simulink model "modular"  (R2013a)
settings: Solver=ode45  StartTime=0.0  StopTime=10.0  RelTol=1e-3
libraries: gated_decay_choice x1, range_choice x1, synaptic_scaling_choice x1
settings Model: Creator=Leo  LastModifiedBy=Leo

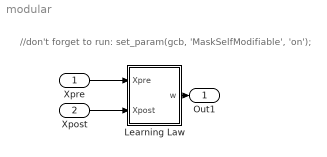
== system modular ==
  note: //don't forget to run:
      | set_param(gcb, 'MaskSelfModifiable', 'on');
  Xpre : Inport
  Xpost : Inport  Port=2
  Learning Law : Subsystem  mask{gorch_y_n=on, gated_decay=Dual OR, multdiv=Divide, synscale=Vanilla Oja, gorch_range=0, lambda1=1, lambda2=0, lambda3=0, lambda4=0, w_0=0, w0=0, alpha1=0, alpha2=0, beta=0, equ=lambda2*[Xpre*Xpost*(gorchrange)+ lambda1*(w_0-w) / ((alpha1*Xpre+alpha2*Xpost^2)*(w-w_0)) + .5lambda3*lambda4*(w_0 - w)comp(w_0,w)*(g(Xpost) - |g(Xpost)|)(g(Xpost))], extr=dg(X)/dt = s-AX, g(0) = -t, comp(w0,w) = |w0-w| <= range}
      mask prompts: gorch_y_n "Would you like a Gorch range?"; gated_decay "What kind of gated decay do you want"; multdiv "Multiply or Divide by the Gated Decay"; synscale "Synaptic Scaling"; gorch_range "Gorch Range"; lambda1 "Learning Rate (1) - Stability"; lambda2 "Learning Rate (2) - Total"; lambda3 "Learning Rate (3, Oja Specific) - Increment"; lambda4 "Learning Rate (4, Oja Specific) - Decrement"; w_0 "Range"; w0 "Initial weight"; alpha1 "Alpha 1 (Additional Parameter)"; alpha2 "Alpha 2 (Additional Parameter)"; beta "Beta (Gorch Gating Term)"; equ "Equation"; extr "Extra info"
      mask help: Make sure to hit apply after selecting your Law Type before moving on to the Law Parameters Tab.
      mask init:
      | eqw ='lambda2*[';
      | dab = gcb;
      | set_param(dab,'extr','');
      | currentVis = get_param(dab,'MaskVisibilities');
      | currentVis{12} = 'off';
      | currentVis{13} = 'off';
      | currentVis{14} = 'off';
      | 
      | if(gorch_y_n)
      |     set_param([dab '/Range'], 'BlockChoice', 'Gorch_range');
      |     currentVis{5} = 'on';
      |     eqw = [eqw 'Xpre*Xpost*(gorchrange)'];
      | else
      |     set_param([dab '/Range'], 'BlockChoice', 'Simple');
      |     currentVis{5} = 'off';
      |     eqw = [eqw 'Xpre*Xpost'];
      | end
      | 
      | eqw = [eqw '+ lambda1*(w_0-w)']
      | 
      | switch multdiv
      |     case 1 %'Multiply'
      |         set_param([dab '/TimesOrDivide'],'Inputs','**');
      |         eqw = [eqw ' * '];
      |     case 2 %'Divide'
      |         set_param([dab '/TimesOrDivide'],'Inputs','*/');
      |         eqw = [eqw ' / '];
      |     case 3 %'Inverse Divide'
      |         set_param([dab '/TimesOrDivide'],'Inputs','/*');
      |         eqw = [eqw ' \ '];
      | end
      | 
      | switch gated_decay
      |     case 1 %'Xpre'
      |         set_param([dab '/Gated Decay Choice'], 'BlockChoice', 'X_pre');
      |         eqw = [eqw 'Xpre'];
      |     case 2 %'Xpost'
      |         set_param([dab '/Gated Decay Choice'], 'BlockChoice', 'X_post');
      |         eqw = [eqw 'Xpost'];
      |     case 3 %'Gorch'
      |         set_param([dab '/Gated Decay Choice'], 'BlockChoice', 'Gorch_Gating');
      |         eqw = [eqw '(Xpost^2 * beta)'];
      |         currentVis{14} = 'on';
      |     case 4 %'Oja'
      |         set_param([dab '/Gated Decay Choice'], 'BlockChoice', 'Oja_Gating');
      |         eqw = [eqw '(Xpost^2*(w-w_0))'];
      |         currentVis{14} = 'off';
      |     case 5 %'Dual OR'
      |         set_param([dab '/Gated Decay Choice'], 'BlockChoice', 'Dual_OR');
      |         eqw = [eqw '((alpha1*Xpre+alpha2*Xpost^2)*(w-w_0))'];
      |         currentVis{12} = 'on';
      |         currentVis{13} = 'on';
      |     case 6 %'Dual AND'
      |         set_param([dab '/Gated Decay Choice'], 'BlockChoice', 'Dual_AND');
      |         eqw = [eqw '(alpha1*Xpre*Xpost^2*(w-w_0))'];
      |         currentVis{12} = 'on';
      | end
      | 
      | switch synscale
      |     case 1 %none
      |         set_param([dab '/Synaptic Scaling Choice'], 'BlockChoice', 'None');
      |         currentVis{8} = 'off';
      |         currentVis{9} = 'off';
      |         eqw = [eqw ']']
      |     case 2 %oja
      |         set_param([dab '/Synaptic Scaling Choice'], 'BlockChoice', 'Oja_stock');
      |         currentVis{8} = 'on';
      |         currentVis{9} = 'on';
      |         eqw = [eqw ' + .5lambda3*lambda4*(w_0 - w)comp(w_0,w)*(g(Xpost) - |g(Xpost)|)(g(Xpost))]'];
      |         set_param(dab,'extr','dg(X)/dt = s-AX, g(0) = -t, comp(w0,w) = |w0-w| <= range');
      | end
      | 
      | set_param(dab,'MaskVisibilities',currentVis);
      | set_param(dab,'equ',eqw);
      settings: AttributesFormatString=dw/dt = %<equ>\n%<extr>
      mask TypeOptions gated_decay: Xpre | Xpost | Gorch | Oja | Dual OR | Dual AND
      mask TypeOptions multdiv: Multiply | Divide | Inverse Divide
      mask TypeOptions synscale: None | Vanilla Oja
  Out1 : Outport
  wires:
  Xpre/1 -> Learning Law/1(Xpre)
  Xpost/1 -> Learning Law/2(Xpost)
  Learning Law/1(w) -> Out1/1

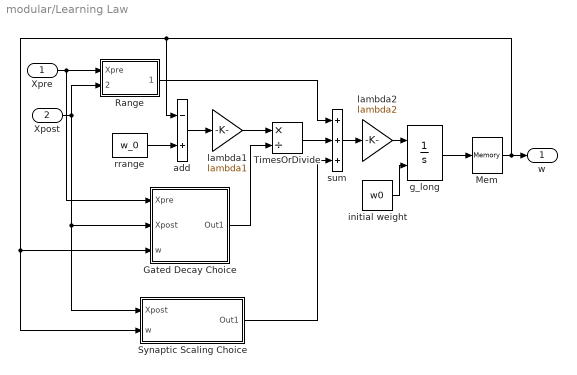
== system modular/Learning Law ==
  Xpre : Inport
  Xpost : Inport  Port=2
  Gated Decay Choice : Subsystem  BlockChoice=Dual_OR
      settings: AttributesFormatString=%<BlockChoice>  TemplateBlock=gated_decay_choice/Gated Decay Choice  MemberBlocks=Dual_AND,Dual_OR,Gorch_Gating,Oja_Gating,X_post,X_pre
  Mem : Memory
  Range : Subsystem  BlockChoice=Gorch_range
      link override Gorch_range/range: Value=gorch_range
      settings: AttributesFormatString=%<BlockChoice>  TemplateBlock=range_choice/Range  MemberBlocks=Gorch_range,Simple
  Synaptic Scaling Choice : Subsystem  BlockChoice=Oja_stock
      settings: AttributesFormatString=%<BlockChoice>  TemplateBlock=synaptic_scaling_choice/Synaptic Scaling Choice  MemberBlocks=None,Oja_stock
  TimesOrDivide : Product  Inputs=*/
  add : Sum  Inputs=-+
  g_long : Integrator  InitialConditionSource=external  ZeroCross=off
  initial weight : Constant  Value=w0
  lambda1 : Gain  Gain=lambda1
  lambda2 : Gain  Gain=lambda2
  rrange : Constant  Value=w_0
  sum : Sum  Inputs=+++
  w : Outport
  wires:
  Xpre/1 -> Range/1(Xpre), Gated Decay Choice/1(Xpre)
  Xpost/1 -> Gated Decay Choice/2(Xpost), Synaptic Scaling Choice/1(Xpost), Range/2(Xpost)
  rrange/1 -> add/2
  Range/1(Out1) -> sum/1
  add/1 -> lambda1/1
  lambda1/1 -> TimesOrDivide/1
  TimesOrDivide/1 -> sum/2
  g_long/1 -> Mem/1
  initial weight/1 -> g_long/2
  Mem/1 -> Synaptic Scaling Choice/2(w), Gated Decay Choice/3(w), add/1, w/1
  Gated Decay Choice/1(Out1) -> TimesOrDivide/2
  lambda2/1 -> g_long/1
  sum/1 -> lambda2/1
  Synaptic Scaling Choice/1(Out1) -> sum/3

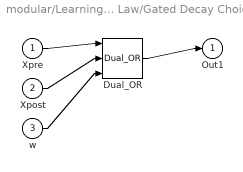
== system modular/Learning Law/Gated Decay Choice ==
  Xpre : Inport
  Xpost : Inport  Port=2
  w : Inport  Port=3
  Dual_OR : gated_decay_choice/Dual_OR
  Out1 : Outport
  wires:
  Xpre/1 -> Dual_OR/1
  Xpost/1 -> Dual_OR/2
  w/1 -> Dual_OR/3
  Dual_OR/1 -> Out1/1

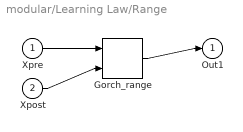
== system modular/Learning Law/Range ==
  Xpre : Inport
  Xpost : Inport  Port=2
  Gorch_range : range_choice/Gorch_range
  Out1 : Outport
  wires:
  Xpre/1 -> Gorch_range/1
  Xpost/1 -> Gorch_range/2
  Gorch_range/1 -> Out1/1

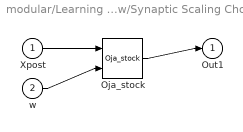
== system modular/Learning Law/Synaptic Scaling Choice ==
  Xpost : Inport
  w : Inport  Port=2
  Oja_stock : synaptic_scaling_choice/Oja_stock
  Out1 : Outport
  wires:
  Xpost/1 -> Oja_stock/1
  w/1 -> Oja_stock/2
  Oja_stock/1 -> Out1/1
